simulink model "simulinkModel"  (R2018b)
settings: Solver=FixedStepAuto  StartTime=0.0  StopTime=1  FixedStep=1E-6  MaxStep=1  MinStep=1E-5  RelTol=1E-3
settings Model: Creator=terab  LastModifiedBy=terab
settings SolverCC: InitialStep=1E-5
settings HardwareCC: ProdBitPerLong=64  ProdLargestAtomicFloat=None  ProdHWDeviceType=AMD->Athlon 64

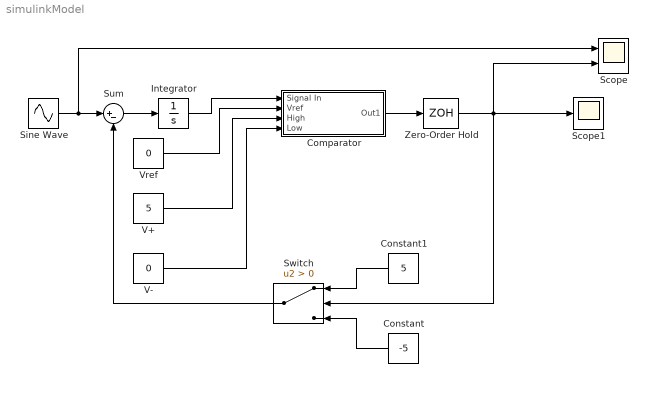
== system simulinkModel ==
  Comparator : Subsystem
  Constant : Constant  Value=-5  VectorParams1D=off
  Constant1 : Constant  Value=5
  Integrator : Integrator
  Scope : Scope  NumInputPorts=2
  Scope1 : Scope
  Sine Wave : Sin  Frequency=2*pi*1000  SampleTime=0
  Sum : Sum  Inputs=|+-
  Switch : Switch  Criteria=u2 > Threshold
  V+ : Constant  Value=5
  V- : Constant  Value=0
  Vref : Constant  Value=0
  Zero-Order Hold : ZeroOrderHold  SampleTime=1E-6
  wires:
  Sine Wave/1 -> Scope/1, Sum/1
  Sum/1 -> Integrator/1
  Constant/1 -> Switch/3
  Constant1/1 -> Switch/1
  Switch/1 -> Sum/2
  Comparator/1(Out1) -> Zero-Order Hold/1
  Integrator/1 -> Comparator/1(Signal In)
  Zero-Order Hold/1 -> Scope1/1, Switch/2, Scope/2
  Vref/1 -> Comparator/2(Vref)
  V+/1 -> Comparator/3(High)
  V-/1 -> Comparator/4(Low)

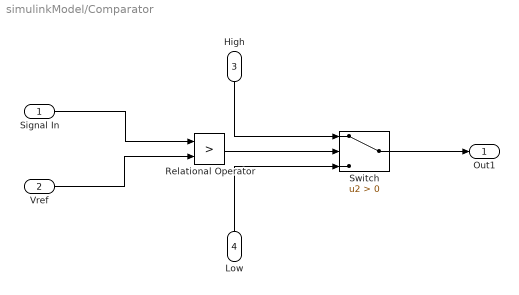
== system simulinkModel/Comparator ==
  Signal In : Inport
  Vref : Inport  Port=2
  High : Inport  Port=3
  Low : Inport  Port=4
  Relational Operator : RelationalOperator  Operator=>  OutDataTypeStr=boolean  RndMeth=Simplest
  Switch : Switch  Criteria=u2 > Threshold
  Out1 : Outport
  wires:
  Signal In/1 -> Relational Operator/1
  Vref/1 -> Relational Operator/2
  Relational Operator/1 -> Switch/2
  High/1 -> Switch/1
  Low/1 -> Switch/3
  Switch/1 -> Out1/1
